simulink model "half_adder"  (R2018a)
settings: Solver=VariableStepAuto  StartTime=0.0  StopTime=10.0  RelTol=1e-3
settings Model: Creator=Edoardo Debenedetti  LastModifiedBy=Edoardo Debenedetti

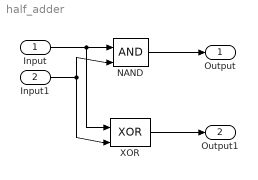
== system half_adder ==
  Input : Inport
  Input1 : Inport  Port=2
  NAND : Logic  IconShape=distinctive  AllPortsSameDT=off  OutDataTypeStr=boolean
  XOR : Logic  Operator=XOR  IconShape=distinctive  AllPortsSameDT=off  OutDataTypeStr=boolean
  Output : Outport
  Output1 : Outport  Port=2
  wires:
  Input/1 -> XOR/1, NAND/1
  XOR/1 -> Output1/1
  NAND/1 -> Output/1
  Input1/1 -> XOR/2, NAND/2
